simulink library "ddm"  (R2021b)
settings: Solver=VariableStepAuto  StartTime=0.0  StopTime=10.0  RelTol=1e-3
undefined symbols (not defined in the file or in its folder): ENUM_ADASACCSTA_ERROR, ENUM_ADASACCSTA_OFF, ENUM_ADASACCSTA_STANDBY, ENUM_ADASISASTA_OFF, ENUM_ALLOWMOV_ALLOWREADY, ENUM_APS, ENUM_BRKSTA_ERROR, ENUM_BRKSTA_OFF, ENUM_BRKSTA_ON, ENUM_CHGPREACTERRSTA_OBCPRE, ENUM_DCDCFAULTSTA_ANYFAULTLV1, ENUM_DCDCFAULTSTA_ANYFAULTLV2, ENUM_DRIVETRAIN_AWD, ENUM_DRIVETRAIN_FWD, ENUM_DRIVETRAIN_RWD, ENUM_DRSEATSTA_INVALID, ENUM_EDUDRTSTA_NORMAL, ENUM_EPBSTA_APPLIED, ENUM_EPBSTA_RELEASED, ENUM_HVBATTREADYPRE_READY, ENUM_MCUWARN_LV0, ENUM_MCUWARN_LV1, ENUM_MCUWARN_LV2, ENUM_MCUWARN_LV3, ENUM_MCUWARN_NOERROR, ENUM_OBCFAULTSTA_ANYFAULT, ENUM_PAS_R2F2, ENUM_PDFAULT_BATTPDFAIL, ENUM_PDFAULT_DCDCDISABLE, ENUM_PDFAULT_MCUDISABLE, ENUM_PDFAULT_MCUDISCHRG, ENUM_POWERSTA_OFF, ENUM_POWERSTA_ON, ENUM_POWERSTA_READY, ENUM_POWERSTA_STANDBY, ENUM_PRESSINDI_LOW, ENUM_PUFAULT_BATTUPFAIL, ENUM_PUFAULT_DCDCENABLEFAIL, ENUM_PUFAULT_PRECHRGCHKFAIL, ENUM_PUFAULT_SAFETYCHKFAIL, ENUM_PUSTATE_COMPLETED, ENUM_PWRSTASW_OFF, ENUM_PWRSTASW_OFFA, ENUM_PWRSTASW_OFFCHVCHRG, ENUM_PWRSTASW_OFFCLVCHRG, ENUM_PWRSTASW_ON, ENUM_PWRSTASW_ONHVCHRG, ENUM_PWRSTASW_READY, ENUM_PWRSTASW_STANDBY, ENUM_RANGESTA_12IN, ENUM_RANGESTA_12OUT, ENUM_SHIFTCOMMAND_D, ENUM_SHIFTCOMMAND_N, ENUM_SHIFTCOMMAND_P, ENUM_SHIFTCOMMAND_R, ENUM_ZONEMALFUNLV_1ST, ENUM_ZONEMALFUNLV_2ND, ENUM_ZONEMALFUNLV_3RD, ENUM_ZONEMALFUNLV_4TH, ENUM_ZONESPDCTRLMODE_ACC ... (+832)
libraries: hcu_lib x738, $bdroot x26, simulink x7
(part 3 of 25)

== system ddm/DDM/DDM/APM ==
  VAPM_USSStaFCL_flg : Inport
  VAPM_USSStaFML_flg : Inport  Port=2
  VAPM_USSStaFMR_flg : Inport  Port=3
  VAPM_USSStaFCR_flg : Inport  Port=4
  VAPM_USSStaRCL_flg : Inport  Port=5
  VAPM_USSStaRML_flg : Inport  Port=6
  VAPM_USSStaRMR_flg : Inport  Port=7
  VAPM_USSStaRCR_flg : Inport  Port=8
  VAPM_USSStaFLL_flg : Inport  Port=9
  VAPM_USSStaFLR_flg : Inport  Port=10
  VAPM_USSStaRLL_flg : Inport  Port=11
  VAPM_USSStaRLR_flg : Inport  Port=12
  DTC_clear_request : Inport  Port=13
  VPMM_SysPwrSta_enum : Inport  Port=14
  VAPM_SNSRLayout_enum : Inport  Port=15
  DTC_Info{,1..11} (12 alike) : hcu_lib/Basic_Blocks/DTC_Info
  Ground{,1..11} (12 alike) : Ground
  Subsystem : Subsystem
  Subsystem1 : Subsystem
  Subsystem{2,4,7..11} (7 alike) : $bdroot/DDM/DDM/APM/Subsystem1  SystemSampleTime=-1  VariantActivationTime=update diagram  Latency=0  AutoFrameSizeCalculation=off
  Subsystem3 : $bdroot/DDM/DDM/APM/Subsystem  SystemSampleTime=-1  VariantActivationTime=update diagram  Latency=0  AutoFrameSizeCalculation=off
  Subsystem5 : $bdroot/DDM/DDM/APM/Subsystem  SystemSampleTime=-1  VariantActivationTime=update diagram  Latency=0  AutoFrameSizeCalculation=off
  Subsystem6 : $bdroot/DDM/DDM/APM/Subsystem  SystemSampleTime=-1  VariantActivationTime=update diagram  Latency=0  AutoFrameSizeCalculation=off
  VDDM_FCLUSSDTC_raw32 : Outport
  VDDM_FMLUSSDTC_raw32 : Outport  Port=2
  VDDM_FMRUSSDTC_raw32 : Outport  Port=3
  VDDM_FCRUSSDTC_raw32 : Outport  Port=4
  VDDM_RCLUSSDTC_raw32 : Outport  Port=5
  VDDM_RMLUSSDTC_raw32 : Outport  Port=6
  VDDM_RMRUSSDTC_raw32 : Outport  Port=7
  VDDM_RCRUSSDTC_raw32 : Outport  Port=8
  VDDM_FLLUSSDTC_raw32 : Outport  Port=9
  VDDM_FLRUSSDTC_raw32 : Outport  Port=10
  VDDM_RLLUSSDTC_raw32 : Outport  Port=11
  VDDM_RLRUSSDTC_raw32 : Outport  Port=12
  wires:
  VAPM_USSStaRLR_flg/1 -> Subsystem11/1
  [VPMM_SysPwrSta_enum] -> Subsystem11/2
  VAPM_USSStaRLL_flg/1 -> Subsystem10/1
  [VPMM_SysPwrSta_enum] -> Subsystem10/2
  VAPM_USSStaFLR_flg/1 -> Subsystem9/1
  [VPMM_SysPwrSta_enum] -> Subsystem9/2
  VAPM_USSStaFLL_flg/1 -> Subsystem8/1
  [VPMM_SysPwrSta_enum] -> Subsystem8/2
  VAPM_USSStaRCR_flg/1 -> Subsystem7/1
  [VPMM_SysPwrSta_enum] -> Subsystem7/2
  VAPM_USSStaRMR_flg/1 -> Subsystem6/1
  [VPMM_SysPwrSta_enum] -> Subsystem6/2
  VAPM_USSStaRML_flg/1 -> Subsystem5/1
  [VPMM_SysPwrSta_enum] -> Subsystem5/2
  VAPM_USSStaRCL_flg/1 -> Subsystem4/1
  [VPMM_SysPwrSta_enum] -> Subsystem4/2
  VAPM_USSStaFCR_flg/1 -> Subsystem3/1
  [VPMM_SysPwrSta_enum] -> Subsystem3/2
  [VPMM_SysPwrSta_enum] -> Subsystem1/2(VPMM_SysPwrSta_enum)
  VPMM_SysPwrSta_enum/1 -> [VPMM_SysPwrSta_enum]
  [VPMM_SysPwrSta_enum] -> Subsystem/2(VPMM_SysPwrSta_enum)
  Subsystem1/2(CFS_flg) -> DTC_Info1/3
  Subsystem1/1(Pass_flg) -> DTC_Info1/2
  Subsystem/2(CFS_flg) -> DTC_Info/3
  Subsystem/1(Pass_flg) -> DTC_Info/2
  VAPM_USSStaFCL_flg/1 -> Subsystem/1(USSSta_flg)
  DTC_Info11/1 -> VDDM_RLRUSSDTC_raw32/1  "VDDM_RLRUSSDTC_raw32"
  Ground11/1 -> DTC_Info11/1
  Ground10/1 -> DTC_Info10/1
  DTC_Info10/1 -> VDDM_RLLUSSDTC_raw32/1  "VDDM_RLLUSSDTC_raw32"
  DTC_Info9/1 -> VDDM_FLRUSSDTC_raw32/1  "VDDM_FLRUSSDTC_raw32"
  Ground8/1 -> DTC_Info8/1
  DTC_Info8/1 -> VDDM_FLLUSSDTC_raw32/1  "VDDM_FLLUSSDTC_raw32"
  DTC_Info7/1 -> VDDM_RCRUSSDTC_raw32/1  "VDDM_RCRUSSDTC_raw32"
  Ground7/1 -> DTC_Info7/1
  Ground6/1 -> DTC_Info6/1
  DTC_Info6/1 -> VDDM_RMRUSSDTC_raw32/1  "VDDM_RMRUSSDTC_raw32"
  DTC_Info5/1 -> VDDM_RMLUSSDTC_raw32/1  "VDDM_RMLUSSDTC_raw32"
  Ground5/1 -> DTC_Info5/1
  DTC_Info4/1 -> VDDM_RCLUSSDTC_raw32/1  "VDDM_RCLUSSDTC_raw32"
  DTC_Info3/1 -> VDDM_FCRUSSDTC_raw32/1  "VDDM_FCRUSSDTC_raw32"
  Ground3/1 -> DTC_Info3/1
  Ground2/1 -> DTC_Info2/1
  DTC_Info2/1 -> VDDM_FMRUSSDTC_raw32/1  "VDDM_FMRUSSDTC_raw32"
  DTC_Info1/1 -> VDDM_FMLUSSDTC_raw32/1  "VDDM_FMLUSSDTC_raw32"
  Ground1/1 -> DTC_Info1/1
  VAPM_USSStaFML_flg/1 -> Subsystem1/1(USSSta_flg)
  [DTC_clear_request] -> DTC_Info1/4
  [DTC_clear_request] -> DTC_Info/4
  DTC_clear_request/1 -> [DTC_clear_request]
  Ground/1 -> DTC_Info/1
  DTC_Info/1 -> VDDM_FCLUSSDTC_raw32/1  "VDDM_FCLUSSDTC_raw32"
  VAPM_SNSRLayout_enum/1 -> [VAPM_SNSRLayout_enum]
  [VAPM_SNSRLayout_enum] -> Subsystem/3(VAPM_SNSRLayout_enum)
  [VAPM_SNSRLayout_enum] -> Subsystem1/3(VAPM_SNSRLayout_enum)
  Subsystem2/1 -> DTC_Info2/2
  Subsystem2/2 -> DTC_Info2/3
  VAPM_USSStaFMR_flg/1 -> Subsystem2/1
  [VPMM_SysPwrSta_enum] -> Subsystem2/2
  [DTC_clear_request] -> DTC_Info2/4
  [VAPM_SNSRLayout_enum] -> Subsystem2/3
  Subsystem3/1 -> DTC_Info3/2
  Subsystem3/2 -> DTC_Info3/3
  [DTC_clear_request] -> DTC_Info3/4
  [VAPM_SNSRLayout_enum] -> Subsystem3/3
  Ground4/1 -> DTC_Info4/1
  Subsystem4/1 -> DTC_Info4/2
  Subsystem4/2 -> DTC_Info4/3
  [DTC_clear_request] -> DTC_Info4/4
  [VAPM_SNSRLayout_enum] -> Subsystem4/3
  Subsystem5/1 -> DTC_Info5/2
  Subsystem5/2 -> DTC_Info5/3
  [DTC_clear_request] -> DTC_Info5/4
  [VAPM_SNSRLayout_enum] -> Subsystem5/3
  Subsystem6/1 -> DTC_Info6/2
  Subsystem6/2 -> DTC_Info6/3
  [DTC_clear_request] -> DTC_Info6/4
  [VAPM_SNSRLayout_enum] -> Subsystem6/3
  Subsystem7/1 -> DTC_Info7/2
  Subsystem7/2 -> DTC_Info7/3
  [DTC_clear_request] -> DTC_Info7/4
  [VAPM_SNSRLayout_enum] -> Subsystem7/3
  Subsystem8/1 -> DTC_Info8/2
  Subsystem8/2 -> DTC_Info8/3
  [DTC_clear_request] -> DTC_Info8/4
  [VAPM_SNSRLayout_enum] -> Subsystem8/3
  Ground9/1 -> DTC_Info9/1
  Subsystem9/1 -> DTC_Info9/2
  Subsystem9/2 -> DTC_Info9/3
  [DTC_clear_request] -> DTC_Info9/4
  [VAPM_SNSRLayout_enum] -> Subsystem9/3
  Subsystem10/1 -> DTC_Info10/2
  Subsystem10/2 -> DTC_Info10/3
  [DTC_clear_request] -> DTC_Info10/4
  [VAPM_SNSRLayout_enum] -> Subsystem10/3
  Subsystem11/1 -> DTC_Info11/2
  Subsystem11/2 -> DTC_Info11/3
  [DTC_clear_request] -> DTC_Info11/4
  [VAPM_SNSRLayout_enum] -> Subsystem11/3

== system ddm/DDM/DDM/BCM ==
  VBCM_DiagHCrash_flg : Inport
  VBCM_DiagFLTS_flg : Inport  Port=2
  VBCM_DiagFRTS_flg : Inport  Port=3
  VBCM_DiagRLTS_flg : Inport  Port=4
  VBCM_DiagRRTS_flg : Inport  Port=5
  DTC_clear_request : Inport  Port=6
  DTC_Info{,1..4} (5 alike) : hcu_lib/Basic_Blocks/DTC_Info
  Ground{,1..4} (5 alike) : Ground
  Logical Operator{1..5} (5 alike) : Logic  Operator=NOT  AllPortsSameDT=off  OutDataTypeStr=boolean
  VDDM_DiagHCrashDTC_raw32 : Outport
  VDDM_DiagFLTSDTC_raw32 : Outport  Port=2
  VDDM_DiagFRTSDTC_raw32 : Outport  Port=3
  VDDM_DiagRLTSDTC_raw32 : Outport  Port=4
  VDDM_DiagRRTSDTC_raw32 : Outport  Port=5
  wires:
  DTC_Info/1 -> VDDM_DiagHCrashDTC_raw32/1  "VDDM_DiagHCrashDTC_raw32"
  Ground/1 -> DTC_Info/1
  VBCM_DiagHCrash_flg/1 -> Logical Operator1/1, DTC_Info/3
  Logical Operator1/1 -> DTC_Info/2
  VBCM_DiagFLTS_flg/1 -> Logical Operator2/1, DTC_Info1/3
  Ground1/1 -> DTC_Info1/1
  Logical Operator2/1 -> DTC_Info1/2
  DTC_Info1/1 -> VDDM_DiagFLTSDTC_raw32/1  "VDDM_DiagFLTSDTC_raw32"
  DTC_Info2/1 -> VDDM_DiagFRTSDTC_raw32/1  "VDDM_DiagFRTSDTC_raw32"
  Logical Operator3/1 -> DTC_Info2/2
  Ground2/1 -> DTC_Info2/1
  VBCM_DiagFRTS_flg/1 -> DTC_Info2/3, Logical Operator3/1
  VBCM_DiagRLTS_flg/1 -> Logical Operator4/1, DTC_Info3/3
  Ground3/1 -> DTC_Info3/1
  Logical Operator4/1 -> DTC_Info3/2
  DTC_Info3/1 -> VDDM_DiagRLTSDTC_raw32/1  "VDDM_DiagRLTSDTC_raw32"
  DTC_Info4/1 -> VDDM_DiagRRTSDTC_raw32/1  "VDDM_DiagRRTSDTC_raw32"
  Logical Operator5/1 -> DTC_Info4/2
  Ground4/1 -> DTC_Info4/1
  VBCM_DiagRRTS_flg/1 -> DTC_Info4/3, Logical Operator5/1
  DTC_clear_request/1 -> [DTC_clear_request]
  [DTC_clear_request] -> DTC_Info2/4
  [DTC_clear_request] -> DTC_Info3/4
  [DTC_clear_request] -> DTC_Info4/4
  [DTC_clear_request] -> DTC_Info1/4
  [DTC_clear_request] -> DTC_Info/4

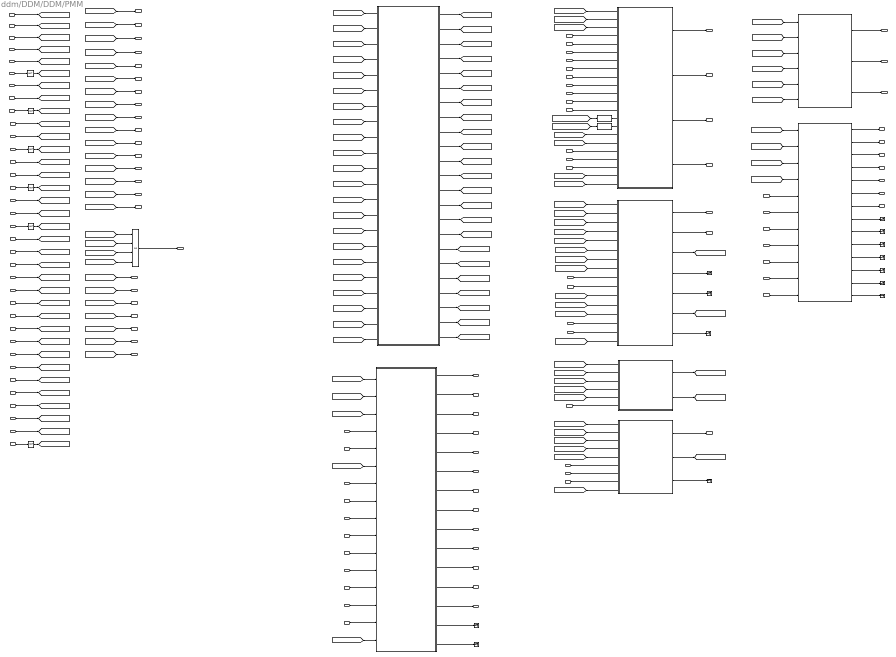
== system ddm/DDM/DDM/PMM ==
  task_time_s : Inport
  VINP_CANMsgValidABM1_flg : Inport  Port=2
  VINP_BrkPedalPosSta_enum : Inport  Port=3
  VINP_BrkPedalPos_pct : Inport  Port=4
  VINP_BrkSWSta_flg : Inport  Port=5
  VINP_CANMsgValidBMS1_flg : Inport  Port=6
  VINP_CANMsgValidBMS6_flg : Inport  Port=7
  VINP_CANMsgValidCCU1_flg : Inport  Port=8
  VINP_CANMsgValidCCU2_flg : Inport  Port=9
  VINP_BMSWarn1_flg : Inport  Port=10
  VINP_BMSWarn2_flg : Inport  Port=11
  VINP_BMSWarn3_flg : Inport  Port=12
  VINP_BMSWarn4_flg : Inport  Port=13
  VINP_BMSWarn5_flg : Inport  Port=14
  VINP_BMSWarn6_flg : Inport  Port=15
  VINP_BMSWarn7_flg : Inport  Port=16
  VINP_BMSWarn8_flg : Inport  Port=17
  VINP_DCDCFaultSta_enum : Inport  Port=18
  VINP_OBCFaultSta_enum : Inport  Port=19
  VINP_MCUWarnF_enum : Inport  Port=20
  VINP_MCUWarnR_enum : Inport  Port=21
  VINP_LVBattDet12V_V : Inport  Port=22
  VINP_BMSREADY_flg : Inport  Port=23
  VINP_HVBattReady4Pre_enum : Inport  Port=24
  VINP_HVBContactorSta_flg : Inport  Port=25
  VINP_DCDCReady4Pre_flg : Inport  Port=26
  VINP_DCDCEnabled_flg : Inport  Port=27
  VINP_CANMsgValidBMS2_flg : Inport  Port=28
  VINP_DrStdAErrSta_enum : Inport  Port=29
  VPMM_PowerSta_enum : Inport  Port=30
  VPMM_PwrStaSW_enum : Inport  Port=31
  VPMM_PowerUpFault_enum : Inport  Port=32
  VPMM_PowerDownFault_enum : Inport  Port=33
  VPMM_DrivetrainSelect_enum : Inport  Port=34
  VPMM_SafetyChkHLv_flg : Inport  Port=35
  VPMM_SafetyChkMLv_flg : Inport  Port=36
  VPMM_HVChrgPreActionErrSta_enum : Inport  Port=37
  VPMM_MCUReady_flg : Inport  Port=38
  VPMM_MCUReady4Pre_flg : Inport  Port=39
  VDDM_C3BMS6RCChk_flg : Inport  Port=40
  VDDM_C3BMS6CSChk_flg : Inport  Port=41
  VDDM_C3BMS1RCChk_flg : Inport  Port=42
  VDDM_C3BMS1CSChk_flg : Inport  Port=43
  VDDM_C3CCU1RCChk_flg : Inport  Port=44
  VDDM_C3CCU1CSChk_flg : Inport  Port=45
  VDDM_C3CCU2RCChk_flg : Inport  Port=46
  VDDM_C3CCU2CSChk_flg : Inport  Port=47
  VDDM_C1ABM1RCChk_flg : Inport  Port=48
  VDDM_C1ABM1CSChk_flg : Inport  Port=49
  VINP_BrakeSWGPIO_flg : Inport  Port=50
  VINP_BrakeLampSW_flg : Inport  Port=51
  VINP_DrStSW : Inport  Port=52
  VINP_FLAJARSW : Inport  Port=53
  VINP_FRAJARSW : Inport  Port=54
  VINP_RLAJARSW : Inport  Port=55
  VINP_RRAJARSW : Inport  Port=56
  VINP_HoodSW : Inport  Port=57
  VINP_TailgaSW : Inport  Port=58
  VDKC_DKCAuthSta_enum : Inport  Port=59
  VINP_AllowMovThd_OTA_enum : Inport  Port=60
  No_CAN1_BUS_OFF : Inport  Port=61
  No_CAN3_BUS_OFF : Inport  Port=62
  VDHP_EAPS12RangeSta_enum : Inport  Port=63
  DTC_clear_request : Inport  Port=64
  VDDM_MCUF1NoComCFS_flg : Inport  Port=65
  VDDM_MCUR1NoComCFS_flg : Inport  Port=66
  VDDM_ESC5NoComCFS_flg : Inport  Port=67
  VDDM_ESC5RCErrCFS_flg : Inport  Port=68
  VDDM_ESC5CSErrCFS_flg : Inport  Port=69
  VDDM_ESC7NoComCFS_flg : Inport  Port=70
  VDDM_ESC7RCErrCFS_flg : Inport  Port=71
  VDDM_ESC7CSErrCFS_flg : Inport  Port=72
  VPMM_PowerUpState_enum : Inport  Port=73
  VINP_CANMsgValidEPAS2_flg : Inport  Port=74
  Brake switch signal abnormal : Subsystem
  Comm err : Subsystem
  Data Type Conversion16 : DataTypeConversion  OutDataTypeStr=boolean
  Data Type Conversion49 : DataTypeConversion  OutDataTypeStr=boolean
  Fault level : Subsystem
  Key authentication failed : Subsystem
  LV : Subsystem
  Logical Operator{,1..4,6} (6 alike) : Logic  Operator=NOT  AllPortsSameDT=off  OutDataTypeStr=boolean
  Logical Operator5 : Logic  Operator=OR  Inputs=4  AllPortsSameDT=off  OutDataTypeStr=boolean
  SW failure : Subsystem
  System conditions of ON to READY not satisfied : Subsystem
  Terminator{,1..12} (13 alike) : Terminator
  power up and power down : Subsystem
  VDDM_C3BMS6RCDTC_raw32 : Outport
  VDDM_C3BMS6CSDTC_raw32 : Outport  Port=2
  VDDM_C3BMS6LCDTC_raw32 : Outport  Port=3
  VDDM_C3BMS1RCDTC_raw32 : Outport  Port=4
  VDDM_C3BMS1CSDTC_raw32 : Outport  Port=5
  VDDM_C3BMS1LCDTC_raw32 : Outport  Port=6
  VDDM_C3CCU1RCDTC_raw32 : Outport  Port=7
  VDDM_C3CCU1CSDTC_raw32 : Outport  Port=8
  VDDM_C3CCU1LCDTC_raw32 : Outport  Port=9
  VDDM_C3CCU2RCDTC_raw32 : Outport  Port=10
  VDDM_C3CCU2CSDTC_raw32 : Outport  Port=11
  VDDM_C3CCU2LCDTC_raw32 : Outport  Port=12
  VDDM_C1ABM1RCDTC_raw32 : Outport  Port=13
  VDDM_C1ABM1CSDTC_raw32 : Outport  Port=14
  VDDM_C1ABM1LCDTC_raw32 : Outport  Port=15
  VDDM_Lv1ErrDTC_raw32 : Outport  Port=16
  VDDM_Lv2ErrDTC_raw32 : Outport  Port=17
  VDDM_Lv3ErrDTC_raw32 : Outport  Port=18
  VDDM_Lv4ErrDTC_raw32 : Outport  Port=19
  VDDM_BrkSWErrDTC_raw32 : Outport  Port=20
  VDDM_BrkSWNoBacDTC_raw32 : Outport  Port=21
  VDDM_KeyAuthDTC_raw32 : Outport  Port=22
  VDDM_ONtoRdyDTC_raw32 : Outport  Port=23
  VDDM_HVB4PreDTC_raw32 : Outport  Port=24
  VDDM_MCU4PreDTC_raw32 : Outport  Port=25
  VDDM_DCDC4PreDTC_raw32 : Outport  Port=26
  VDDM_HVRlyCloDTC_raw32 : Outport  Port=27
  VDDM_BMSRdyDTC_raw32 : Outport  Port=28
  VDDM_DCDCEnaDTC_raw32 : Outport  Port=29
  VDDM_HiLvSaChkDTC_raw32 : Outport  Port=30
  VDDM_MidLvSaChkDTC_raw32 : Outport  Port=31
  VDDM_MCUDisDTC_raw32 : Outport  Port=32
  VDDM_DCDCDisDTC_raw32 : Outport  Port=33
  VDDM_HVRlyOpDTC_raw32 : Outport  Port=34
  VDDM_MCUActDTC_raw32 : Outport  Port=35
  VDDM_OBC4PreDTC_raw32 : Outport  Port=36
  VDDM_IniLVLoDTC_raw32 : Outport  Port=37
  VDDM_LVSupLoDTC_raw32 : Outport  Port=38
  VDDM_LVSupHiDTC_raw32 : Outport  Port=39
  VDDM_DrStSWDTC_raw32 : Outport  Port=40
  VDDM_FLDoorSWDTC_raw32 : Outport  Port=41
  VDDM_RLDoorSWDTC_raw32 : Outport  Port=42
  VDDM_FRDoorSWDTC_raw32 : Outport  Port=43
  VDDM_RRDoorSWDTC_raw32 : Outport  Port=44
  VDDM_HoodSWDTC_raw32 : Outport  Port=45
  VDDM_TailgaSWDTC_raw32 : Outport  Port=46
  VDDM_EDriveSysErrPMM_flg : Outport  Port=47
  VDDM_C3BMS6CSCFS_flg : Outport  Port=48
  VDDM_C3BMS6RCCFS_flg : Outport  Port=49
  VDDM_C3BMS6LCCFS_flg : Outport  Port=50
  VDDM_C3CCU2CSCFS_flg : Outport  Port=51
  VDDM_C3CCU2LCCFS_flg : Outport  Port=52
  VDDM_C3CCU2RCCFS_flg : Outport  Port=53
  VDDM_C1EPAS2LCDTC_raw32 : Outport  Port=54
  wires:
  VINP_BMSWarn4_flg/1 -> Fault level/7(VINP_BMSWarn4_flg)
  VINP_CANMsgValidABM1_flg/1 -> Logical Operator4/1
  [VDDM_C3BMS6LCChk_flg] -> Comm err/6(VDDM_C3BMS6LCChk_flg)
  VINP_BMSWarn1_flg/1 -> Fault level/4(VINP_BMSWarn1_flg)
  Logical Operator2/1 -> [VDDM_C3CCU1LCChk_flg]
  VINP_CANMsgValidBMS6_flg/1 -> Logical Operator/1
  VINP_BMSWarn5_flg/1 -> Fault level/8(VINP_BMSWarn5_flg)
  VINP_BMSWarn2_flg/1 -> Fault level/5(VINP_BMSWarn2_flg)
  VINP_CANMsgValidBMS1_flg/1 -> Logical Operator1/1
  [VDDM_C3BMS1CSChk_flg] -> Comm err/8(VDDM_C3BMS1CSChk_flg)
  VINP_BMSWarn8_flg/1 -> Fault level/11(VINP_BMSWarn8_flg)
  No_CAN1_BUS_OFF/1 -> [No_CAN1_BUS_OFF]
  task_time_s/1 -> [task_time_s]
  VINP_BrkSWSta_flg/1 -> Brake switch signal abnormal/10(VINP_BrkSWSta_flg)
  [VDDM_C3BMS1LCChk_flg] -> Comm err/9(VDDM_C3BMS1LCChk_flg)
  [VINP_BrakeSWGPIO_flg] -> Brake switch signal abnormal/4(VINP_BrakeSWGPIO_flg)
  [VDDM_C3CCU2RCChk_flg] -> Comm err/13(VDDM_C3CCU2RCChk_flg)
  [VPMM_PwrStaSW_enum] -> Brake switch signal abnormal/2(VPMM_PwrStaSW_enum)
  VINP_BrkPedalPos_pct/1 -> Brake switch signal abnormal/15(VINP_BrkPedalPos_pct)
  [VPMM_PwrStaSW_enum] -> Fault level/2(VPMM_PwrStaSW_enum)
  VPMM_DrivetrainSelect_enum/1 -> Fault level/13(VPMM_DrivetrainSelect_enum)
  VDDM_C3CCU2CSChk_flg/1 -> [VDDM_C3CCU2CSChk_flg]
  VDDM_C3CCU1CSChk_flg/1 -> [VDDM_C3CCU1CSChk_flg]
  [task_time_s] -> Key authentication failed/1(task_time_s)
  [DTC_clear_request] -> Key authentication failed/5(DTC_clear_request)
  Logical Operator/1 -> [VDDM_C3BMS6LCChk_flg]
  VDDM_C3BMS6RCChk_flg/1 -> [VDDM_C3BMS6RCChk_flg]
  [VPMM_PowerSta_enum] -> SW failure/3(VPMM_PowerSta_enum)
  VINP_OBCFaultSta_enum/1 -> Fault level/20(VINP_OBCFaultSta_enum)
  [DTC_clear_request] -> Comm err/21(DTC_clear_request)
  [task_time_s] -> Brake switch signal abnormal/1(task_time_s)
  [VPMM_PwrStaSW_enum] -> power up and power down/2(VPMM_PwrStaSW_enum)
  [task_time_s] -> SW failure/1(task_time_s)
  VINP_DCDCEnabled_flg/1 -> power up and power down/12(VINP_DCDCEnabled_flg)
  VINP_MCUWarnF_enum/1 -> Fault level/18(VINP_MCUWarnF_enum)
  [No_CAN3_BUS_OFF] -> Comm err/19(No_CAN3_BUS_OFF)
  [VDDM_ESC5NoComCFS_flg] -> Brake switch signal abnormal/6(VDDM_ESC5NoComCFS_flg)
  [VDDM_C3BMS6RCChk_flg] -> Comm err/4(VDDM_C3BMS6RCChk_flg)
  [VPMM_PwrStaSW_enum] -> SW failure/2(VPMM_PwrStaSW_enum)
  VINP_BrakeSWGPIO_flg/1 -> [VINP_BrakeSWGPIO_flg]
  VDDM_C3BMS6CSChk_flg/1 -> [VDDM_C3BMS6CSChk_flg]
  [VINP_BrakeLampSW_flg] -> Brake switch signal abnormal/5(VINP_BrakeLampSW_flg)
  VINP_FLAJARSW/1 -> SW failure/6(VINP_FLAJARSW)
  Brake switch signal abnormal/6(VDDM_EDriveSysErrBrake_flg) -> [VDDM_EDriveSysErrBrake_flg]
  [VDDM_C3BMS6CSChk_flg] -> Comm err/5(VDDM_C3BMS6CSChk_flg)
  VINP_FRAJARSW/1 -> SW failure/7(VINP_FRAJARSW)
  [VPMM_PowerSta_enum] -> Fault level/3(VPMM_PowerSta_enum)
  VINP_BrkPedalPosSta_enum/1 -> Brake switch signal abnormal/14(VINP_BrkPedalPosSta_enum)
  [task_time_s] -> Fault level/1(task_time_s)
  VINP_BMSWarn3_flg/1 -> Fault level/6(VINP_BMSWarn3_flg)
  VDDM_C3CCU1RCChk_flg/1 -> [VDDM_C3CCU1RCChk_flg]
  VPMM_HVChrgPreActionErrSta_enum/1 -> power up and power down/15(VPMM_HVChrgPreActionErrSta_enum)
  [VPMM_PowerSta_enum] -> Brake switch signal abnormal/3(VPMM_PowerSta_enum)
  VINP_BrakeLampSW_flg/1 -> [VINP_BrakeLampSW_flg]
  [VDDM_C3CCU2CSChk_flg] -> Comm err/14(VDDM_C3CCU2CSChk_flg)
  Comm err/16(VDDM_EDriveSysErrABMCAN_flg) -> [VDDM_EDriveSysErrABMCAN_flg]
  [task_time_s] -> Comm err/1(task_time_s)
  VINP_LVBattDet12V_V/1 -> [VINP_LVBattDet12V_V]
  Brake switch signal abnormal/3(VDDM_BrakeSW_enum) -> [VDDM_BrakeSW_enum]
  [VPMM_PwrStaSW_enum] -> LV/2(VPMM_PwrStaSW_enum)
  Logical Operator3/1 -> [VDDM_C3CCU2LCChk_flg]
  VINP_DCDCFaultSta_enum/1 -> Fault level/12(VINP_DCDCFaultSta_enum)
  [VDDM_C3BMS1RCChk_flg] -> Comm err/7(VDDM_C3BMS1RCChk_flg)
  VDDM_C1ABM1CSChk_flg/1 -> [VDDM_C1ABM1CSChk_flg]
  [VPMM_PowerSta_enum] -> power up and power down/3(VPMM_PowerSta_enum)
  [VDDM_C3CCU1CSChk_flg] -> Comm err/11(VDDM_C3CCU1CSChk_flg)
  [task_time_s] -> LV/1(task_time_s)
  [task_time_s] -> power up and power down/1(task_time_s)
  VDDM_C3CCU2RCChk_flg/1 -> [VDDM_C3CCU2RCChk_flg]
  [VDDM_C1ABM1LCChk_flg] -> Comm err/18(VDDM_C1ABM1LCChk_flg)
  VDKC_DKCAuthSta_enum/1 -> Key authentication failed/6(VDKC_DKCAuthSta_enum)
  [DTC_clear_request] -> power up and power down/6(DTC_clear_request)
  [VPMM_PwrStaSW_enum] -> Comm err/3(VPMM_PwrStaSW_enum)
  [VDDM_BrakeSW_enum] -> Key authentication failed/4(VDDM_BrakeSW_enum)
  [VPMM_PwrStaSW_enum] -> System conditions of ON to READY not satisfied/2(VPMM_PowerSta_enum)
  VINP_AllowMovThd_OTA_enum/1 -> System conditions of ON to READY not satisfied/7(VINP_AllowMovThd_OTA_enum)
  [VPMM_PowerSta_enum] -> Key authentication failed/3(VPMM_PwrStaSW_enum)
  VINP_MCUWarnR_enum/1 -> Fault level/19(VINP_MCUWarnR_enum)
  VPMM_PwrStaSW_enum/1 -> [VPMM_PwrStaSW_enum]
  [VDDM_C3CCU1LCChk_flg] -> Comm err/12(VDDM_C3CCU1LCChk_flg)
  Logical Operator1/1 -> [VDDM_C3BMS1LCChk_flg]
  VDDM_C3BMS1RCChk_flg/1 -> [VDDM_C3BMS1RCChk_flg]
  VINP_CANMsgValidBMS2_flg/1 -> [VINP_CANMsgValidBMS2_flg]
  VPMM_PowerUpFault_enum/1 -> power up and power down/4(VPMM_PowerUpFault_enum)
  VPMM_PowerDownFault_enum/1 -> power up and power down/5(VPMM_PowerDownFault_enum)
  VINP_HVBattReady4Pre_enum/1 -> power up and power down/7(VINP_HVBattReady4Pre_enum)
  [VDDM_EDriveSysErrABMCAN_flg] -> Logical Operator5/1
  VPMM_SafetyChkHLv_flg/1 -> power up and power down/13(VPMM_SafetyChkHLv_flg)
  VINP_DCDCReady4Pre_flg/1 -> power up and power down/9(VINP_DCDCReady4Pre_flg)
  [No_CAN1_BUS_OFF] -> Comm err/20(No_CAN1_BUS_OFF)
  VDHP_EAPS12RangeSta_enum/1 -> System conditions of ON to READY not satisfied/8(VDHP_EAPS12RangeSta_enum)
  VINP_BMSWarn7_flg/1 -> Fault level/10(VINP_BMSWarn7_flg)
  VPMM_MCUReady4Pre_flg/1 -> power up and power down/8(VPMM_MCUReady4Pre_flg)
  VDDM_C1ABM1RCChk_flg/1 -> [VDDM_C1ABM1RCChk_flg]
  [VDDM_BrakeSW_enum] -> System conditions of ON to READY not satisfied/4(VDDM_BrakeSW_enum)
  [VDDM_C1ABM1CSChk_flg] -> Comm err/17(VDDM_C1ABM1CSChk_flg)
  [VDDM_ESC7NoComCFS_flg] -> Brake switch signal abnormal/11(VDDM_ESC7NoComCFS_flg)
  [VDDM_C3CCU2LCChk_flg] -> Comm err/15(VDDM_C3CCU2LCChk_flg)
  [VINP_CANMsgValidBMS2_flg] -> LV/5(VINP_CANMsgValidBMS2_flg)
  Logical Operator4/1 -> [VDDM_C1ABM1LCChk_flg]
  Logical Operator5/1 -> VDDM_EDriveSysErrPMM_flg/1  "VDDM_EDriveSysErrVCUErr_flg"
  Key authentication failed/2(VDDM_EDriveSysErrKeyAuth_flg) -> [VDDM_EDriveSysErrKeyAuth_flg]
  [task_time_s] -> System conditions of ON to READY not satisfied/1(task_time_s)
  [VDDM_ESC5CSErrCFS_flg] -> Brake switch signal abnormal/8(VDDM_ESC5CSErrCFS_flg)
  VINP_HVBContactorSta_flg/1 -> power up and power down/10(VINP_HVBContactorSta_flg)
  VPMM_PowerSta_enum/1 -> [VPMM_PowerSta_enum]
  [VDDM_EDriveSysErrKeyAuth_flg] -> Logical Operator5/4
  [VDDM_ESC7CSErrCFS_flg] -> Brake switch signal abnormal/13(VDDM_ESC7CSErrCFS_flg)
  [VDDM_C1ABM1RCChk_flg] -> Comm err/16(VDDM_C1ABM1RCChk_flg)
  VINP_CANMsgValidCCU2_flg/1 -> Logical Operator3/1
  [DTC_clear_request] -> System conditions of ON to READY not satisfied/5(DTC_clear_request)
  VPMM_MCUReady_flg/1 -> System conditions of ON to READY not satisfied/6(VPMM_MCUReady_flg)
  VINP_RRAJARSW/1 -> SW failure/9(VINP_RRAJARSW)
  VINP_DrStSW/1 -> SW failure/5(VINP_DrStSW)
  VPMM_SafetyChkMLv_flg/1 -> power up and power down/14(VPMM_SafetyChkMLv_flg)
  [VDDM_C3CCU1RCChk_flg] -> Comm err/10(VDDM_C3CCU1RCChk_flg)
  VINP_BMSWarn6_flg/1 -> Fault level/9(VINP_BMSWarn6_flg)
  [VDDM_ESC7RCErrCFS_flg] -> Brake switch signal abnormal/12(VDDM_ESC7RCErrCFS_flg)
  [DTC_clear_request] -> SW failure/4(DTC_clear_request)
  [VPMM_PowerSta_enum] -> LV/3(VPMM_PowerSta_enum)
  [VPMM_PowerSta_enum] -> Comm err/2(VPMM_PowerSta_enum)
  VINP_BMSREADY_flg/1 -> power up and power down/11(VINP_BMSREADY_flg)
  VINP_DrStdAErrSta_enum/1 -> Brake switch signal abnormal/9(VINP_DrStdAErrSta_enum)
  [VDDM_MCUR1NoComCFS_flg] -> Fault level/17(VDDM_MCUR1NoComCFS_flg)
  VINP_HoodSW/1 -> SW failure/10(VINP_HoodSW)
  [VDDM_KeyAuthDTC_raw32] -> System conditions of ON to READY not satisfied/9(VDDM_KeyAuthDTC_raw32)
  [VDDM_EDriveSysErrONtoRdy_flg] -> Logical Operator5/2
  [VDDM_ESC5RCErrCFS_flg] -> Brake switch signal abnormal/7(VDDM_ESC5RCErrCFS_flg)
  DTC_clear_request/1 -> [DTC_clear_request]
  [VDDM_MCUF1NoComCFS_flg] -> Fault level/16(VDDM_MCUF1NoComCFS_flg)
  [DTC_clear_request] -> LV/6(DTC_clear_request)
  [VDDM_EDriveSysErrBrake_flg] -> Logical Operator5/3
  VDDM_C3BMS1CSChk_flg/1 -> [VDDM_C3BMS1CSChk_flg]
  No_CAN3_BUS_OFF/1 -> [No_CAN3_BUS_OFF]
  [VINP_LVBattDet12V_V] -> LV/4(VINP_LVBattDet12V_V)
  VINP_RLAJARSW/1 -> SW failure/8(VINP_RLAJARSW)
  [DTC_clear_request] -> Brake switch signal abnormal/16(DTC_clear_request)
  VINP_TailgaSW/1 -> SW failure/11(VINP_TailgaSW)
  System conditions of ON to READY not satisfied/2(VDDM_EDriveSysErrONtoRdy_flg) -> [VDDM_EDriveSysErrONtoRdy_flg]
  [VPMM_PowerSta_enum] -> System conditions of ON to READY not satisfied/3(VPMM_PwrStaSW_enum)
  VINP_CANMsgValidCCU1_flg/1 -> Logical Operator2/1
  [VPMM_PwrStaSW_enum] -> Key authentication failed/2(VPMM_PowerSta_enum)
  Comm err/1(VDDM_C3BMS6RCDTC_raw32) -> [VDDM_C3BMS6RCDTC_raw32]
  Comm err/2(VDDM_C3BMS6CSDTC_raw32) -> [VDDM_C3BMS6CSDTC_raw32]
  Comm err/3(VDDM_C3BMS6LCDTC_raw32) -> [VDDM_C3BMS6LCDTC_raw32]
  Comm err/4(VDDM_C3BMS1RCDTC_raw32) -> [VDDM_C3BMS1RCDTC_raw32]
  Comm err/5(VDDM_C3BMS1CSDTC_raw32) -> [VDDM_C3BMS1CSDTC_raw32]
  Comm err/6(VDDM_C3BMS1LCDTC_raw32) -> [VDDM_C3BMS1LCDTC_raw32]
  Comm err/7(VDDM_C3CCU1RCDTC_raw32) -> [VDDM_C3CCU1RCDTC_raw32]
  Comm err/8(VDDM_C3CCU1CSDTC_raw32) -> [VDDM_C3CCU1CSDTC_raw32]
  Comm err/9(VDDM_C3CCU1LCDTC_raw32) -> [VDDM_C3CCU1LCDTC_raw32]
  Comm err/10(VDDM_C3CCU2RCDTC_raw32) -> [VDDM_C3CCU2RCDTC_raw32]
  Comm err/11(VDDM_C3CCU2CSDTC_raw32) -> [VDDM_C3CCU2CSDTC_raw32]
  Comm err/12(VDDM_C3CCU2LCDTC_raw32) -> [VDDM_C3CCU2LCDTC_raw32]
  Comm err/13(VDDM_C1ABM1RCDTC_raw32) -> [VDDM_C1ABM1RCDTC_raw32]
  Comm err/14(VDDM_C1ABM1CSDTC_raw32) -> [VDDM_C1ABM1CSDTC_raw32]
  Comm err/15(VDDM_C1ABM1LCDTC_raw32) -> [VDDM_C1ABM1LCDTC_raw32]
  [VDDM_C3BMS1CSDTC_raw32] -> VDDM_C3BMS1CSDTC_raw32/1
  [VDDM_C3BMS1LCDTC_raw32] -> VDDM_C3BMS1LCDTC_raw32/1
  [VDDM_C3CCU1RCDTC_raw32] -> VDDM_C3CCU1RCDTC_raw32/1
  [VDDM_C3CCU1CSDTC_raw32] -> VDDM_C3CCU1CSDTC_raw32/1
  [VDDM_C3CCU1LCDTC_raw32] -> VDDM_C3CCU1LCDTC_raw32/1
  [VDDM_C3CCU2RCDTC_raw32] -> VDDM_C3CCU2RCDTC_raw32/1
  [VDDM_C3CCU2CSDTC_raw32] -> VDDM_C3CCU2CSDTC_raw32/1
  [VDDM_C3CCU2LCDTC_raw32] -> VDDM_C3CCU2LCDTC_raw32/1
  [VDDM_C1ABM1RCDTC_raw32] -> VDDM_C1ABM1RCDTC_raw32/1
  [VDDM_C1ABM1CSDTC_raw32] -> VDDM_C1ABM1CSDTC_raw32/1
  [VDDM_C1ABM1LCDTC_raw32] -> VDDM_C1ABM1LCDTC_raw32/1
  LV/1(VDDM_IniLVLoDTC_raw32) -> VDDM_IniLVLoDTC_raw32/1
  LV/2(VDDM_LVSupLoDTC_raw32) -> VDDM_LVSupLoDTC_raw32/1
  LV/3(VDDM_LVSupHiDTC_raw32) -> VDDM_LVSupHiDTC_raw32/1
  Brake switch signal abnormal/1(VDDM_BrkSWErrDTC_raw32) -> VDDM_BrkSWErrDTC_raw32/1
  Brake switch signal abnormal/2(VDDM_BrkSWNoBacDTC_raw32) -> VDDM_BrkSWNoBacDTC_raw32/1
  Fault level/1(VDDM_Lv1ErrDTC_raw32) -> VDDM_Lv1ErrDTC_raw32/1
  System conditions of ON to READY not satisfied/1(VDDM_ONtoRdyDTC_raw32) -> VDDM_ONtoRdyDTC_raw32/1
  [VDDM_C3BMS6RCDTC_raw32] -> VDDM_C3BMS6RCDTC_raw32/1
  [VDDM_C3BMS1RCDTC_raw32] -> VDDM_C3BMS1RCDTC_raw32/1
  [VDDM_C3BMS6LCDTC_raw32] -> VDDM_C3BMS6LCDTC_raw32/1
  [VDDM_C3BMS6CSDTC_raw32] -> VDDM_C3BMS6CSDTC_raw32/1
  power up and power down/2(VDDM_MCU4PreDTC_raw32) -> VDDM_MCU4PreDTC_raw32/1
  power up and power down/1(VDDM_HVB4PreDTC_raw32) -> VDDM_HVB4PreDTC_raw32/1
  power up and power down/3(VDDM_DCDC4PreDTC_raw32) -> VDDM_DCDC4PreDTC_raw32/1
  power up and power down/4(VDDM_HVRlyCloDTC_raw32) -> VDDM_HVRlyCloDTC_raw32/1
  power up and power down/5(VDDM_BMSRdyDTC_raw32) -> VDDM_BMSRdyDTC_raw32/1
  power up and power down/6(VDDM_DCDCEnaDTC_raw32) -> VDDM_DCDCEnaDTC_raw32/1
  power up and power down/7(VDDM_HiLvSaChkDTC_raw32) -> VDDM_HiLvSaChkDTC_raw32/1
  power up and power down/8(VDDM_MidLvSaChkDTC_raw32) -> VDDM_MidLvSaChkDTC_raw32/1
  power up and power down/9(VDDM_MCUDisDTC_raw32) -> VDDM_MCUDisDTC_raw32/1
  power up and power down/10(VDDM_DCDCDisDTC_raw32) -> VDDM_DCDCDisDTC_raw32/1
  power up and power down/11(VDDM_HVRlyOpDTC_raw32) -> VDDM_HVRlyOpDTC_raw32/1
  power up and power down/12(VDDM_MCUActDTC_raw32) -> VDDM_MCUActDTC_raw32/1
  power up and power down/13(VDDM_OBC4PreDTC_raw32) -> VDDM_OBC4PreDTC_raw32/1
  SW failure/1(VDDM_DrStSWDTC_raw32) -> VDDM_DrStSWDTC_raw32/1
  SW failure/2(VDDM_FLDoorSWDTC_raw32) -> VDDM_FLDoorSWDTC_raw32/1
  SW failure/3(VDDM_RLDoorSWDTC_raw32) -> VDDM_RLDoorSWDTC_raw32/1
  SW failure/4(VDDM_FRDoorSWDTC_raw32) -> VDDM_FRDoorSWDTC_raw32/1
  SW failure/5(VDDM_RRDoorSWDTC_raw32) -> VDDM_RRDoorSWDTC_raw32/1
  SW failure/6(VDDM_HoodSWDTC_raw32) -> VDDM_HoodSWDTC_raw32/1
  SW failure/7(VDDM_TailgaSWDTC_raw32) -> VDDM_TailgaSWDTC_raw32/1
  SW failure/8(Dr_SeatSta) -> Terminator/1
  SW failure/14(VCUTailgaSWSta) -> Terminator6/1
  SW failure/9(VCUFLDoorSta) -> Terminator1/1
  SW failure/10(VCUFRDoorSta) -> Terminator2/1
  SW failure/11(VCURLDoorSta) -> Terminator3/1
  SW failure/12(VCURRDoorSta) -> Terminator4/1
  SW failure/13(VCUHoodSWSta) -> Terminator5/1
  power up and power down/14(VDDM_HVRlyOpFail_flg) -> Terminator7/1
  power up and power down/15(VDDM_MCUActDisFail_flg) -> Terminator8/1
  System conditions of ON to READY not satisfied/3(VDDM_SysAllowReadySta_flg) -> Terminator9/1
  Brake switch signal abnormal/4(VDDM_CANBrkSW2Sta_enum) -> Terminator10/1
  Brake switch signal abnormal/5(VDDM_BrkPedalPosSta_enum) -> Terminator11/1
  Brake switch signal abnormal/7(VDDM_VCUBrkSWSta_flg) -> Terminator12/1
  Key authentication failed/1(VDDM_KeyAuthDTC_raw32) -> [VDDM_KeyAuthDTC_raw32]
  [VDDM_KeyAuthDTC_raw32] -> VDDM_KeyAuthDTC_raw32/1
  VDDM_MCUF1NoComCFS_flg/1 -> [VDDM_MCUF1NoComCFS_flg]
  VDDM_MCUR1NoComCFS_flg/1 -> [VDDM_MCUR1NoComCFS_flg]
  VDDM_ESC5NoComCFS_flg/1 -> [VDDM_ESC5NoComCFS_flg]
  VDDM_ESC5RCErrCFS_flg/1 -> [VDDM_ESC5RCErrCFS_flg]
  VDDM_ESC5CSErrCFS_flg/1 -> [VDDM_ESC5CSErrCFS_flg]
  VDDM_ESC7NoComCFS_flg/1 -> [VDDM_ESC7NoComCFS_flg]
  VDDM_ESC7RCErrCFS_flg/1 -> [VDDM_ESC7RCErrCFS_flg]
  VDDM_ESC7CSErrCFS_flg/1 -> [VDDM_ESC7CSErrCFS_flg]
  Fault level/2(VDDM_Lv2ErrCFS_flg) -> VDDM_Lv2ErrDTC_raw32/1
  Fault level/3(VDDM_Lv3ErrDTC_raw32) -> VDDM_Lv3ErrDTC_raw32/1
  Fault level/4(VDDM_Lv4ErrDTC_raw32) -> VDDM_Lv4ErrDTC_raw32/1
  [VDDM_C3BMS6LCDTC_raw32] -> Data Type Conversion49/1
  [DTC_clear_request] -> Fault level/21(DTC_clear_request)
  [No_CAN3_BUS_OFF] -> Fault level/22(No_CAN3_BUS_OFF)
  Data Type Conversion49/1 -> Fault level/14(VDDM_C3BMS6LCCFS_flg)
  [VDDM_C3CCU2LCDTC_raw32] -> Data Type Conversion16/1
  Data Type Conversion16/1 -> Fault level/15(VDDM_C3CCU2LCCFS_flg)
  VPMM_PowerUpState_enum/1 -> [VPMM_PowerUpState_enum]
  [VPMM_PowerUpState_enum] -> power up and power down/16(VPMM_PowerUpState_enum)
  Comm err/17(VDDM_C3BMS6CSCFS_flg) -> [VDDM_C3BMS6CSCFS_flg]
  Comm err/18(VDDM_C3BMS6RCCFS_flg) -> [VDDM_C3BMS6RCCFS_flg]
  Comm err/19(VDDM_C3BMS6LCCFS_flg) -> [VDDM_C3BMS6LCCFS_flg]
  Comm err/20(VDDM_C3CCU2CSCFS_flg) -> [VDDM_C3CCU2CSCFS_flg]
  Comm err/21(VDDM_C3CCU2LCCFS_flg) -> [VDDM_C3CCU2LCCFS_flg]
  Comm err/22(VDDM_C3CCU2RCCFS_flg) -> [VDDM_C3CCU2RCCFS_flg]
  [VDDM_C3BMS6CSCFS_flg] -> VDDM_C3BMS6CSCFS_flg/1
  [VDDM_C3BMS6RCCFS_flg] -> VDDM_C3BMS6RCCFS_flg/1
  [VDDM_C3BMS6LCCFS_flg] -> VDDM_C3BMS6LCCFS_flg/1
  [VDDM_C3CCU2CSCFS_flg] -> VDDM_C3CCU2CSCFS_flg/1
  [VDDM_C3CCU2LCCFS_flg] -> VDDM_C3CCU2LCCFS_flg/1
  [VDDM_C3CCU2RCCFS_flg] -> VDDM_C3CCU2RCCFS_flg/1
  Comm err/23(VDDM_C1EPAS2LCDTC_raw32) -> [VDDM_C1EPAS2LCDTC_raw32]
  [VDDM_C1EPAS2LCChk_flg] -> Comm err/22(VDDM_C1EPAS2LCChk_flg)
  VINP_CANMsgValidEPAS2_flg/1 -> Logical Operator6/1
  Logical Operator6/1 -> [VDDM_C1EPAS2LCChk_flg]
  [VDDM_C1EPAS2LCDTC_raw32] -> VDDM_C1EPAS2LCDTC_raw32/1

== system ddm/DDM/DDM/TPM ==
  note: SensorFail
  note: WheelTmpHigh
  note: PressureLow
  note: Batwarn
  task_time_s : Inport
  VPMM_PowerSta_enum : Inport  Port=2
  DTC_clear_request : Inport  Port=3
  VTPM_LFBatwarn_flg : Inport  Port=4
  VTPM_RFBatwarn_flg : Inport  Port=5
  VTPM_LRBatwarn_flg : Inport  Port=6
  VTPM_RRBatwarn_flg : Inport  Port=7
  VTPM_LFPressIndi_enum : Inport  Port=8
  VTPM_RFPressIndi_enum : Inport  Port=9
  VTPM_LRPressIndi_enum : Inport  Port=10
  VTPM_RRPressIndi_enum : Inport  Port=11
  VTPM_LFWheelTmpIndi_flg : Inport  Port=12
  VTPM_RFWheelTmpIndi_flg : Inport  Port=13
  VTPM_LRWheelTmpIndi_flg : Inport  Port=14
  VTPM_RRWheelTmpIndi_flg : Inport  Port=15
  VTPM_LFSensorFail_flg : Inport  Port=16
  VTPM_RFSensorFail_flg : Inport  Port=17
  VTPM_LRSensorFail_flg : Inport  Port=18
  VTPM_RRSensorFail_flg : Inport  Port=19
  LFBatwarn : Subsystem
  LFPressureLow : Subsystem
  LFSensorfail : Subsystem
  LFWheelTmpHigh : Subsystem
  LRBatwarn : Subsystem
  LRPressureLow : Subsystem
  LRSensorfail : Subsystem
  LRWheelTmpHigh : Subsystem
  RFBatwarn : Subsystem
  RFPressureLow : Subsystem
  RFSensorfail : Subsystem
  RFWheelTmpHigh : Subsystem
  RRBatwarn : Subsystem
  RRPressureLow : Subsystem
  RRSensorfail : Subsystem
  RRWheelTmpHigh : Subsystem
  VDDM_LFBatwarnDTC_raw32 : Outport
  VDDM_RFBatwarnDTC_raw32 : Outport  Port=2
  VDDM_LRBatwarnDTC_raw32 : Outport  Port=3
  VDDM_RRBatwarnDTC_raw32 : Outport  Port=4
  VDDM_LFPressIndiDTC_raw32 : Outport  Port=5
  VDDM_RFPressIndiDTC_raw32 : Outport  Port=6
  VDDM_LRPressIndiDTC_raw32 : Outport  Port=7
  VDDM_RRPressIndiDTC_raw32 : Outport  Port=8
  VDDM_LFWheelTmpHighDTC_raw32 : Outport  Port=9
  VDDM_RFWheelTmpHighDTC_raw32 : Outport  Port=10
  VDDM_LRWheelTmpHighDTC_raw32 : Outport  Port=11
  VDDM_RRWheelTmpHighDTC_raw32 : Outport  Port=12
  VDDM_LFSensorFailDTC_raw32 : Outport  Port=13
  VDDM_RFSensorFailDTC_raw32 : Outport  Port=14
  VDDM_LRSensorFailDTC_raw32 : Outport  Port=15
  VDDM_RRSensorFailDTC_raw32 : Outport  Port=16
  wires:
  VPMM_PowerSta_enum/1 -> [VPMM_PowerSta_enum]
  DTC_clear_request/1 -> [DTC_clear_request]
  task_time_s/1 -> [task_time_s]
  [VPMM_PowerSta_enum] -> LFBatwarn/2(VPMM_PowerSta_enum)
  [task_time_s] -> LFBatwarn/1(task_time_s)
  [DTC_clear_request] -> LFBatwarn/3(DTC_clear_request)
  VTPM_LFBatwarn_flg/1 -> LFBatwarn/4(VTPM_LFBatwarn_flg)
  LFBatwarn/1(VDDM_LFBatwarnDTC_raw32) -> VDDM_LFBatwarnDTC_raw32/1
  [task_time_s] -> RFBatwarn/1(task_time_s)
  [VPMM_PowerSta_enum] -> RFBatwarn/2(VPMM_PowerSta_enum)
  [DTC_clear_request] -> RFBatwarn/3(DTC_clear_request)
  VTPM_RFBatwarn_flg/1 -> RFBatwarn/4(VTPM_RFBatwarn_flg)
  RFBatwarn/1(VDDM_RFBatwarnDTC_raw32) -> VDDM_RFBatwarnDTC_raw32/1
  [task_time_s] -> LRBatwarn/1(task_time_s)
  [VPMM_PowerSta_enum] -> LRBatwarn/2(VPMM_PowerSta_enum)
  [DTC_clear_request] -> LRBatwarn/3(DTC_clear_request)
  VTPM_LRBatwarn_flg/1 -> LRBatwarn/4(VTPM_LRBatwarn_flg)
  LRBatwarn/1(VDDM_LRBatwarnDTC_raw32) -> VDDM_LRBatwarnDTC_raw32/1
  RRBatwarn/1(VDDM_RRBatwarnDTC_raw32) -> VDDM_RRBatwarnDTC_raw32/1
  [task_time_s] -> RRBatwarn/1(task_time_s)
  [VPMM_PowerSta_enum] -> RRBatwarn/2(VPMM_PowerSta_enum)
  [DTC_clear_request] -> RRBatwarn/3(DTC_clear_request)
  VTPM_RRBatwarn_flg/1 -> RRBatwarn/4(VTPM_RRBatwarn_flg)
  [task_time_s] -> LFPressureLow/1(task_time_s)
  [VPMM_PowerSta_enum] -> LFPressureLow/2(VPMM_PowerSta_enum)
  [DTC_clear_request] -> LFPressureLow/3(DTC_clear_request)
  [task_time_s] -> RFPressureLow/1(task_time_s)
  [VPMM_PowerSta_enum] -> RFPressureLow/2(VPMM_PowerSta_enum)
  [DTC_clear_request] -> RFPressureLow/3(DTC_clear_request)
  [DTC_clear_request] -> LRPressureLow/3(DTC_clear_request)
  [VPMM_PowerSta_enum] -> LRPressureLow/2(VPMM_PowerSta_enum)
  [task_time_s] -> LRPressureLow/1(task_time_s)
  [task_time_s] -> RRPressureLow/1(task_time_s)
  [VPMM_PowerSta_enum] -> RRPressureLow/2(VPMM_PowerSta_enum)
  [DTC_clear_request] -> RRPressureLow/3(DTC_clear_request)
  LFPressureLow/1(VDDM_LFPressIndiDTC_raw32) -> VDDM_LFPressIndiDTC_raw32/1
  RFPressureLow/1(VDDM_RFPressIndiDTC_raw32) -> VDDM_RFPressIndiDTC_raw32/1
  LRPressureLow/1(VDDM_LRPressIndiDTC_raw32) -> VDDM_LRPressIndiDTC_raw32/1
  RRPressureLow/1(VDDM_RRPressIndiDTC_raw32) -> VDDM_RRPressIndiDTC_raw32/1
  VTPM_LFPressIndi_enum/1 -> LFPressureLow/4(VTPM_LFPressIndi_enum)
  VTPM_RFPressIndi_enum/1 -> RFPressureLow/4(VTPM_RFPressIndi_enum)
  VTPM_LRPressIndi_enum/1 -> LRPressureLow/4(VTPM_LRPressIndi_enum)
  VTPM_RRPressIndi_enum/1 -> RRPressureLow/4(VTPM_RRPressIndi_enum)
  [task_time_s] -> LFWheelTmpHigh/1(task_time_s)
  [VPMM_PowerSta_enum] -> LFWheelTmpHigh/2(VPMM_PowerSta_enum)
  [DTC_clear_request] -> LFWheelTmpHigh/3(DTC_clear_request)
  [task_time_s] -> RFWheelTmpHigh/1(task_time_s)
  [VPMM_PowerSta_enum] -> RFWheelTmpHigh/2(VPMM_PowerSta_enum)
  [DTC_clear_request] -> RFWheelTmpHigh/3(DTC_clear_request)
  [task_time_s] -> LRWheelTmpHigh/1(task_time_s)
  [VPMM_PowerSta_enum] -> LRWheelTmpHigh/2(VPMM_PowerSta_enum)
  [DTC_clear_request] -> LRWheelTmpHigh/3(DTC_clear_request)
  [task_time_s] -> RRWheelTmpHigh/1(task_time_s)
  [VPMM_PowerSta_enum] -> RRWheelTmpHigh/2(VPMM_PowerSta_enum)
  [DTC_clear_request] -> RRWheelTmpHigh/3(DTC_clear_request)
  VTPM_LFWheelTmpIndi_flg/1 -> LFWheelTmpHigh/4(VTPM_LFWheelTmpHigh_flg)
  VTPM_RFWheelTmpIndi_flg/1 -> RFWheelTmpHigh/4(VTPM_RFWheelTmpHigh_flg)
  VTPM_LRWheelTmpIndi_flg/1 -> LRWheelTmpHigh/4(VTPM_LRWheelTmpHigh_flg)
  VTPM_RRWheelTmpIndi_flg/1 -> RRWheelTmpHigh/4(VTPM_RRWheelTmpHigh_flg)
  LFWheelTmpHigh/1(VDDM_LFWheelTmpHighDTC_raw32) -> VDDM_LFWheelTmpHighDTC_raw32/1
  RFWheelTmpHigh/1(VDDM_RFWheelTmpHighDTC_raw32) -> VDDM_RFWheelTmpHighDTC_raw32/1
  LRWheelTmpHigh/1(VDDM_LRWheelTmpHighDTC_raw32) -> VDDM_LRWheelTmpHighDTC_raw32/1
  RRWheelTmpHigh/1(VDDM_RRWheelTmpHighDTC_raw32) -> VDDM_RRWheelTmpHighDTC_raw32/1
  [task_time_s] -> LFSensorfail/1(task_time_s)
  [VPMM_PowerSta_enum] -> LFSensorfail/2(VPMM_PowerSta_enum)
  [DTC_clear_request] -> LFSensorfail/3(DTC_clear_request)
  [task_time_s] -> RFSensorfail/1(task_time_s)
  [VPMM_PowerSta_enum] -> RFSensorfail/2(VPMM_PowerSta_enum)
  [DTC_clear_request] -> RFSensorfail/3(DTC_clear_request)
  [task_time_s] -> LRSensorfail/1(task_time_s)
  [VPMM_PowerSta_enum] -> LRSensorfail/2(VPMM_PowerSta_enum)
  [DTC_clear_request] -> LRSensorfail/3(DTC_clear_request)
  [task_time_s] -> RRSensorfail/1(task_time_s)
  [VPMM_PowerSta_enum] -> RRSensorfail/2(VPMM_PowerSta_enum)
  [DTC_clear_request] -> RRSensorfail/3(DTC_clear_request)
  VTPM_LFSensorFail_flg/1 -> LFSensorfail/4(VTPM_LFSensorFail_flg)
  VTPM_RFSensorFail_flg/1 -> RFSensorfail/4(VTPM_RFSensorFail_flg)
  VTPM_LRSensorFail_flg/1 -> LRSensorfail/4(VTPM_LRSensorFail_flg)
  VTPM_RRSensorFail_flg/1 -> RRSensorfail/4(VTPM_RRSensorFail_flg)
  LFSensorfail/1(VDDM_LFSensorFailDTC_raw32) -> VDDM_LFSensorFailDTC_raw32/1
  RFSensorfail/1(VDDM_RFSensorFailDTC_raw32) -> VDDM_RFSensorFailDTC_raw32/1
  LRSensorfail/1(VDDM_LRSensorFailDTC_raw32) -> VDDM_LRSensorFailDTC_raw32/1
  RRSensorfail/1(VDDM_RRSensorFailDTC_raw32) -> VDDM_RRSensorFailDTC_raw32/1
